simulink model "EMD_model_1"  (R2018b)
settings: Solver=ode45  StartTime=0.0  StopTime=setStopTime  FixedStep=0.0005  RelTol=1e-3  EnableMultiTasking=on
model workspace (MAT data in the model file):
  bodyAmp = 0
  bodyPhase = 0
  freq = 628.318530718
  headAmp = 0
  headPhase = 0
  imageData = [0.00228480667088 0.00685422825671 0.0114230745906 0.0159909622235 0.0205575077854 0.0251223280162 0.0296850397975 0.0342452601838 0.0388026064343 0.0433566960441 0.0479071467754 0.0524535766893 ... (8204 elements, 1x8204)]
  outputTimeList = [1 1.0001 1.0002 1.0003 1.0004 1.0005 1.0006 1.0007 1.0008 1.0009 1.001 1.0011 1.0012 1.0013 1.0014 1.0015 1.0016 1.0017 1.0018 1.0019 1.002 1.0021 1.0022 1.0023 1.0024 1.0025 1.0026 1.0027 1.0028 1.0029 1.003 1.0031 1.0032 1.0033 1.0034 1.0035 1.0036 1.0037 1.0038 1.0039 1.004 1.0041 1.0042 1.0043 1.0044 1.0045 1.0046 1.0047 1.0048 1.0049 1.005 1.0051 1.0052 1.0053 1.0054 1.0055 1.0056 1.0057 1.0058 1.0059 1.006 1.0061 1.0062 1.0063 1.0064 1.0065 1.0066 1.0067 1.0068 1.0069 1.007 1.0071 1.0072 1.0073 1.0074 1.0075 1.0076 1.0077 1.0078 1.0079 1.008 1.0081 1.0082 1.0083 1.0084 1.0085 1.0086 1.0087 1.0088 1.0089 1.009 1.0091 1.0092 1.0093 1.0094 1.0095 1.0096 1.0097 1.0098 1.0099 1.01]
  setStopTime = 1.01
  stimAmp = 15
  temporalFilt = 0.035
  timeConstant = 0.06
undefined symbols (not defined in the file): high_delay, low_delay, phot_a, photo_b
libraries: visionsources x1
(part 1 of 2)
settings Model: SimulationMode=accelerator  Creator=Shane  LastModifiedBy=BC
settings DataIOCC: SaveFormat=Array  ReturnWorkspaceOutputs=on  OutputOption=SpecifiedOutputTimes  OutputTimes=outputTimeList
settings OptimizationCC: ExpressionDepthLimit=2147483647  EfficientMapNaN2IntZero=off  SimCompilerOptimization=on
settings DebuggingCC: UnderspecifiedInitializationDetection=Classic  MergeDetectMultiDrivingBlocksExec=none  FcnCallInpInsideContextMsg=warning  StateNameClashWarn=warning  SFUnexpectedBacktrackingDiag=warning  SFNoUnconditionalDefaultTransitionDiag=warning  SFExecutionAtInitializationDiag=none
settings HardwareCC: ProdBitPerPointer=32  ProdBitPerSizeT=32  ProdBitPerPtrDiffT=32  ProdLargestAtomicFloat=None  ProdIntDivRoundTo=Undefined  ProdEndianess=Unspecified  ProdWordSize=32  ProdHWDeviceType=32-bit Generic  TargetBitPerPointer=64  TargetBitPerSizeT=64  TargetBitPerPtrDiffT=64  TargetLongLongMode=on  TargetIntDivRoundTo=Zero  TargetEndianess=LittleEndian  TargetWordSize=64  TargetHWDeviceType=MATLAB Host  ProdEqTarget=off
settings ModelReferenceCC: PropagateSignalLabelsOutOfModel=off
settings SFSimCC: SimUseLocalCustomCode=off
settings RTWCC: SystemTargetFile=accel.tlc  TemplateMakefile=accel_default_tmf  RTWVerbose=off
settings CodeAppCC: MaxIdLength=128
settings STFCustomTargetCC: ConcurrentExecutionCompliant=on  MATLABClassNameForMDSCustomization=Simulink.SoftwareTarget.TargetSpecificTriggerConfigurationBase  GRTInterface=on  SystemTargetFile=accel.tlc
settings ConfigComp: CovMetricSettings=dw  CovHtmlReporting=on  CovSaveCumulativeToWorkspaceVar=on  CovSaveSingleToWorkspaceVar=on  CovExternalEMLEnable=off

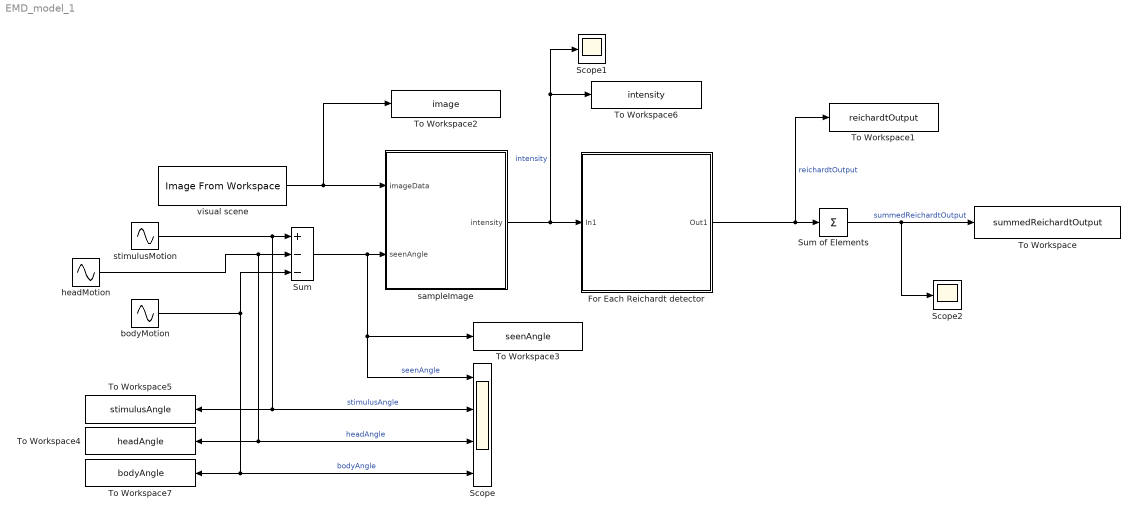
== system EMD_model_1 ==
  For Each Reichardt detector : Subsystem  TreatAsAtomicUnit=on
  Scope : Scope  NumInputPorts=4
  Scope1 : Scope
  Scope2 : Scope
  Sum : Sum  Inputs=+--
  Sum of Elements : Sum  Inputs=+
  To Workspace : ToWorkspace  VariableName=summedReichardtOutput  SaveFormat=Timeseries  SampleTime=-1
  To Workspace1 : ToWorkspace  VariableName=reichardtOutput  SaveFormat=Timeseries  SampleTime=-1
  To Workspace2 : ToWorkspace  VariableName=image  SaveFormat=Timeseries  SampleTime=-1
  To Workspace3 : ToWorkspace  VariableName=seenAngle  SaveFormat=Timeseries  SampleTime=-1
  To Workspace4 : ToWorkspace  VariableName=headAngle  SaveFormat=Timeseries  SampleTime=-1
  To Workspace5 : ToWorkspace  VariableName=stimulusAngle  SaveFormat=Timeseries  SampleTime=-1
  To Workspace6 : ToWorkspace  VariableName=intensity  SaveFormat=Timeseries  SampleTime=-1
  To Workspace7 : ToWorkspace  VariableName=bodyAngle  SaveFormat=Timeseries  SampleTime=-1
  bodyMotion : Sin  Amplitude=bodyAmp  Frequency=freq  Phase=bodyPhase  SampleTime=0
  headMotion : Sin  Amplitude=headAmp  Frequency=freq  Phase=headPhase  SampleTime=0
  sampleImage : MATLAB Function  TreatAsAtomicUnit=on
  stimulusMotion : Sin  Amplitude=stimAmp  Frequency=freq  SampleTime=0
  visual scene : visionsources/Image From Workspace  Tag=vipblks_nd  ImageValue=imageData  Ts=inf  imagePorts=One multidimensional signal  OutPortLabels=R|G|B  ImageDataType=double  Signed=on  WordLength=16  sdImageDataType=sfix(16)  FractionLengthMode=User-defined  FractionLength=15
      settings: SourceProductName=Computer Vision Toolbox  SourceProductBaseCode=VP
  wires:
  For Each Reichardt detector/1(Out1) -> To Workspace1/1, Sum of Elements/1  "reichardtOutput"
  Sum of Elements/1 -> Scope2/1, To Workspace/1  "summedReichardtOutput"
  sampleImage/1(intensity) -> Scope1/1, To Workspace6/1, For Each Reichardt detector/1(In1)  "intensity"
  visual scene/1 -> To Workspace2/1, sampleImage/1(imageData)
  stimulusMotion/1 -> To Workspace5/1, Scope/2, Sum/1  "stimulusAngle"
  headMotion/1 -> To Workspace4/1, Scope/3, Sum/2  "headAngle"
  Sum/1 -> Scope/1, To Workspace3/1, sampleImage/2(seenAngle)  "seenAngle"
  bodyMotion/1 -> Sum/3, To Workspace7/1, Scope/4  "bodyAngle"
